simulink model "modelStandup"  (R2013b)
settings: Solver=ode4  StartTime=0.0  StopTime=tSim  FixedStep=h  RelTol=1e-3
values from neighbouring files (symbols this model uses):
  modelSelect = 'full'    [launcher_script.m]    (also in launcher_simulink.m = 'linear')
  params = [M,m,L,I,b,g]    [launcher_script.m]    (also in launcher_simulink.m)
  state0 = [thetaDot0;theta0;xDot0;x0]    [launcher_script.m]    (also in launcher_simulink.m; sFunction.m = [])
settings Model: Creator=JAR  LastModifiedBy=JAR

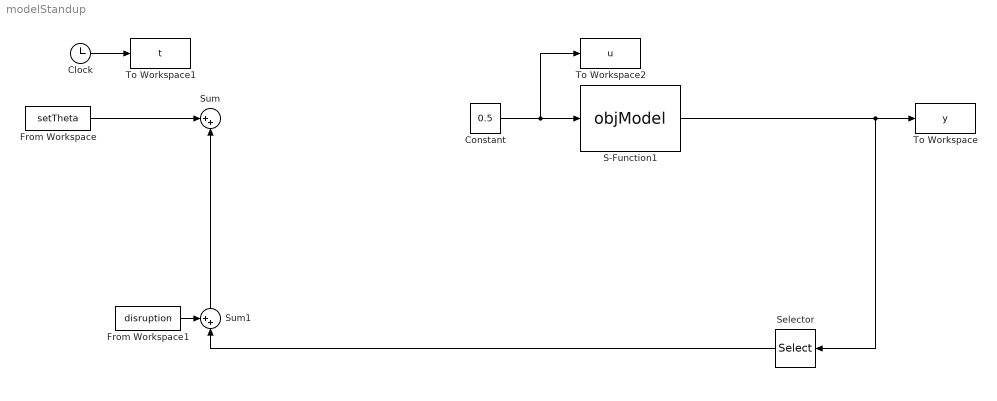
== system modelStandup ==
  Clock : Clock
  Constant : Constant  Value=0.5
  From Workspace : FromWorkspace  VariableName=setTheta  SampleTime=0
  From Workspace1 : FromWorkspace  VariableName=disruption  SampleTime=0
  S-Function1 : S-Function  FunctionName=objModel  Parameters=state0,params,modelSelect  EnableBusSupport=off
  Selector : Selector  InputPortWidth=4  IndexOptions=Index vector (dialog)  Indices=2  OutputSizes=1
  Sum : Sum  Inputs=|++
  Sum1 : Sum  Inputs=++|
  To Workspace : ToWorkspace  VariableName=y  SampleTime=-1
  To Workspace1 : ToWorkspace  VariableName=t  SampleTime=-1
  To Workspace2 : ToWorkspace  VariableName=u  SampleTime=-1
  wires:
  Clock/1 -> To Workspace1/1
  From Workspace1/1 -> Sum1/1
  Sum1/1 -> Sum/2
  Selector/1 -> Sum1/2
  From Workspace/1 -> Sum/1
  Constant/1 -> To Workspace2/1, S-Function1/1
  S-Function1/1 -> Selector/1, To Workspace/1
